simulink model "EffectuatorIntegratedWithDemonstrator"  (R2020a)
settings: Solver=FixedStepDiscrete  StartTime=0.0  StopTime=inf  FixedStep=Ts  RelTol=1e-3
InitFcn:
  | %% Verwende vordefinierte Setpoints (Kreis mit Z-Komponente)
  | 
  | % Config
  | numCircles = 3;
  | scale=6;
  | %Versuch symmetrische Setpunkte zu setzen
  | pointsPerCircle =scale*(4+3*numCircles)+2;
  | 
  | r = 50;
  | m_x = r;
  | m_y = r;
  | 
  | % //
  | s = linspace(0,2*pi,pointsPerCircle);
  | 
  | setPoints_x = [];
  | setPoints_y = [];
  | 
  | for ii=1:numCircles
  | 
  | setPoints_x = [setPoints_x (-cos(s(1:floor(pointsPerCircle / 2))).*r + m_x + 2*r*(ii-1))]; %#ok<AGROW>
  | setPoints_y = [setPoints_y (sin(s).*r+m_y)]; %#ok<AGROW>pointsPerCircle / 2
  | 
  | end
  | 
  | setPoints_x = [setPoints_x flip(setPoints_x(1:end))];
  | 
  | % Loeschen doppelter y-Werte (Kreisuebergang)
  | setPoints_x(pointsPerCircle .* [1:numCircles]) = [];
  | setPoints_y(pointsPerCircle .* [1:numCircles]) = [];
  | 
  | % setPoints_x= [linspace(0,setPoints_x(19),19) setPoints_x(20:end)];
  | % setPoints_y= [linspace(0,setPoints_y(19),19) setPoints_y(20:end)];
  | 
  | % Array Elemente verschieben
  | % setPoints_x = circshift(setPoints_x,-pointsPerCircle/4,2);
  | % setPoints_y = circshift(setPoints_y,-pointsPerCircle/4,2);
  | 
  | z = zeros(1,size(setPoints_x,2));
  | z_x = -5:5;
  | z_y = -z_x.^2 + 25;
  | z_idx = 90;
  | z_idx2 = 210;
  | z(z_idx:z_idx+length(z_x)-1) = z_y;
  | z(z_idx2:z_idx2+length(z_x)-1) = z_y;
  | % z = [z_y z];
  | setPoints_z = z;
  | 
  | % setPoints_x = [zeros(1,length(z_y)) setPoints_x];
  | % setPoints_y = [setPoints_y(1,1)*ones(1,length(z_y)) setPoints_y];
  | 
  | % Umrechnung der Einheiten für Demonstrator
  | % setPoints_x = setPoints_x ./ 1000;
  | % setPoints_y = setPoints_y ./ 1000;
  | % setPoints_z = setPoints_z ./ 1000;
  | 
  | 
  | %{
  | plot(setPoints_x,setPoints_y);
  | fig = figure;
  | ... (+13 lines)
StartFcn:
  | close all;
model workspace (MAT data in the model file):
  MvmtPerfEval_collectVal : Simulink.Parameter (value not decoded)
  MvmtPerfEval_sendOwnVal : Simulink.Parameter (value not decoded)
  PerfEval_numTicks_enable : Simulink.Parameter (value not decoded)
  Segmentregler_I_Gain : Simulink.Parameter (value not decoded)
  Segmentregler_P_Gain : Simulink.Parameter (value not decoded)
  Segmentregler_minVel_enable : Simulink.Parameter (value not decoded)
  Segmentregler_numTicks_enable : Simulink.Parameter (value not decoded)
  Ts : Simulink.Parameter (value not decoded)
  maxPos_x : Simulink.Parameter (value not decoded)
  maxPos_y : Simulink.Parameter (value not decoded)
  maxPos_z : Simulink.Parameter (value not decoded)
  maxVectorLengths : Simulink.Parameter (value not decoded)
  minAllowedVelSaturation : Simulink.Parameter (value not decoded)
  numAxes : Simulink.Parameter (value not decoded)
symbols that are objects in the model workspace (value not decoded): maxPos_x, maxPos_y, maxPos_z, minAllowedVelSaturation, MvmtPerfEval_collectVal, MvmtPerfEval_sendOwnVal, numAxes, PerfEval_numTicks_enable, Segmentregler_I_Gain, Segmentregler_minVel_enable, Segmentregler_numTicks_enable, Segmentregler_P_Gain, Ts
undefined symbols (not defined in the file or in its folder): DiscIntNeverNeededParam, VelOverride
libraries: simulink x20, vrlib x5, sldrtlib x2, xpcrtudplib x2, dspnetwork x2, ptplib x1, etargetslib x1, xpcutilitieslib x1
(part 4 of 5)

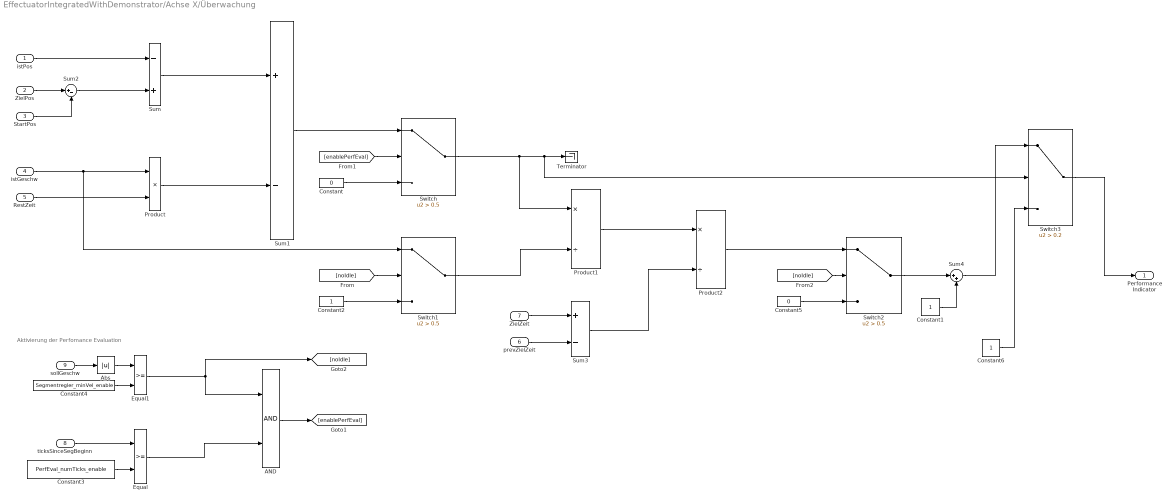
== system EffectuatorIntegratedWithDemonstrator/Achse X/Überwachung ==
  note: Aktivierung der Perfomance Evaluation
  istPos : Inport
  ZielPos : Inport  Port=2
  StartPos : Inport  Port=3
  istGeschw : Inport  Port=4
  RestZeit : Inport  Port=5
  prevZielZeit : Inport  Port=6
  ZielZeit : Inport  Port=7
  ticksSinceSegBeginn : Inport  Port=8
  sollGeschw : Inport  Port=9
  AND : Logic  AllPortsSameDT=off  OutDataTypeStr=boolean
  Abs : Abs
  Constant : Constant  Value=0
  Constant1 : Constant
  Constant2 : Constant
  Constant3 : Constant  Value=PerfEval_numTicks_enable
  Constant4 : Constant  Value=Segmentregler_minVel_enable
  Constant5 : Constant  Value=0
  Constant6 : Constant
  Equal : RelationalOperator  OutDataTypeStr=boolean  RndMeth=Simplest
  Equal1 : RelationalOperator  OutDataTypeStr=boolean  RndMeth=Simplest
  Product : Product
  Product1 : Product  Inputs=*/
  Product2 : Product  Inputs=*/
  Sum : Sum  Inputs=-+
  Sum1 : Sum  Inputs=+-
  Sum2 : Sum  Inputs=|+-
  Sum3 : Sum  Inputs=+-
  Sum4 : Sum  Inputs=|++
  Switch : Switch  Criteria=u2 > Threshold  Threshold=0.5
  Switch1 : Switch  Criteria=u2 > Threshold  Threshold=0.5
  Switch2 : Switch  Criteria=u2 > Threshold  Threshold=0.5
  Switch3 : Switch  Criteria=u2 > Threshold  Threshold=0.2
  Terminator : Terminator
  Performance Indicator : Outport  VectorParamsAs1DForOutWhenUnconnected=off
  wires:
  istPos/1 -> Sum/1
  istGeschw/1 -> Switch1/1, Product/1
  RestZeit/1 -> Product/2
  Product/1 -> Sum1/2
  Sum/1 -> Sum1/1
  ZielPos/1 -> Sum2/1
  StartPos/1 -> Sum2/2
  Sum2/1 -> Sum/2
  Sum1/1 -> Switch/1
  Switch/1 -> Product1/1, Switch3/2, Terminator/1
  [enablePerfEval] -> Switch/2
  Constant/1 -> Switch/3
  Product1/1 -> Product2/1
  Sum3/1 -> Product2/2
  prevZielZeit/1 -> Sum3/2
  ZielZeit/1 -> Sum3/1
  Sum4/1 -> Switch3/1
  Constant1/1 -> Sum4/2
  ticksSinceSegBeginn/1 -> Equal/1
  Constant3/1 -> Equal/2
  Equal/1 -> AND/2
  sollGeschw/1 -> Abs/1
  Constant4/1 -> Equal1/2
  Equal1/1 -> [noIdle], AND/1
  AND/1 -> [enablePerfEval]
  [noIdle] -> Switch1/2
  Constant2/1 -> Switch1/3
  Switch1/1 -> Product1/2
  Switch2/1 -> Sum4/1
  Product2/1 -> Switch2/1
  [noIdle] -> Switch2/2
  Constant5/1 -> Switch2/3
  Abs/1 -> Equal1/1
  Switch3/1 -> Performance Indicator/1
  Constant6/1 -> Switch3/3

== system EffectuatorIntegratedWithDemonstrator/Achse Y/Sat_maxGeschw ==
  Threshold : Inport
  In : Inport  Port=2
  Threshold1 : Inport  Port=3
  Abs : Abs
  Constant : Constant  Value=0
  Multiply : Gain  Gain=-1
  Sign : Signum
  Sum3 : Sum  Inputs=-+
  Switch : Switch  Criteria=u2 > Threshold
  Switch1 : Switch
  Switch2 : Switch  Criteria=u2 > Threshold
  Out : Outport  VectorParamsAs1DForOutWhenUnconnected=off
  wires:
  Sum3/1 -> Switch/2
  Threshold/1 -> Switch/1, Sum3/1
  Abs/1 -> Sum3/2, Switch/3
  In/1 -> Sign/1, Abs/1
  Sign/1 -> Switch1/2
  Switch/1 -> Multiply/1, Switch1/1
  Multiply/1 -> Switch1/3
  Switch2/1 -> Out/1
  Constant/1 -> Switch2/3
  Threshold1/1 -> Switch2/2
  Switch1/1 -> Switch2/1

== system EffectuatorIntegratedWithDemonstrator/Achse Y/Sat_sollGeschw ==
  Threshold : Inport
  In : Inport  Port=2
  Abs : Abs
  Constant : Constant  Value=minAllowedVelSaturation
  Max : MinMax  Function=max  Inputs=2
  Multiply : Gain  Gain=-1
  Sign : Signum
  Sum3 : Sum  Inputs=-+
  Switch : Switch  Criteria=u2 > Threshold
  Switch1 : Switch
  Out : Outport  VectorParamsAs1DForOutWhenUnconnected=off
  wires:
  Constant/1 -> Max/2
  Threshold/1 -> Max/1
  Switch1/1 -> Out/1
  Multiply/1 -> Switch1/3
  Switch/1 -> Switch1/1, Multiply/1
  Sign/1 -> Switch1/2
  In/1 -> Abs/1, Sign/1
  Abs/1 -> Switch/3, Sum3/2
  Max/1 -> Sum3/1, Switch/1
  Sum3/1 -> Switch/2

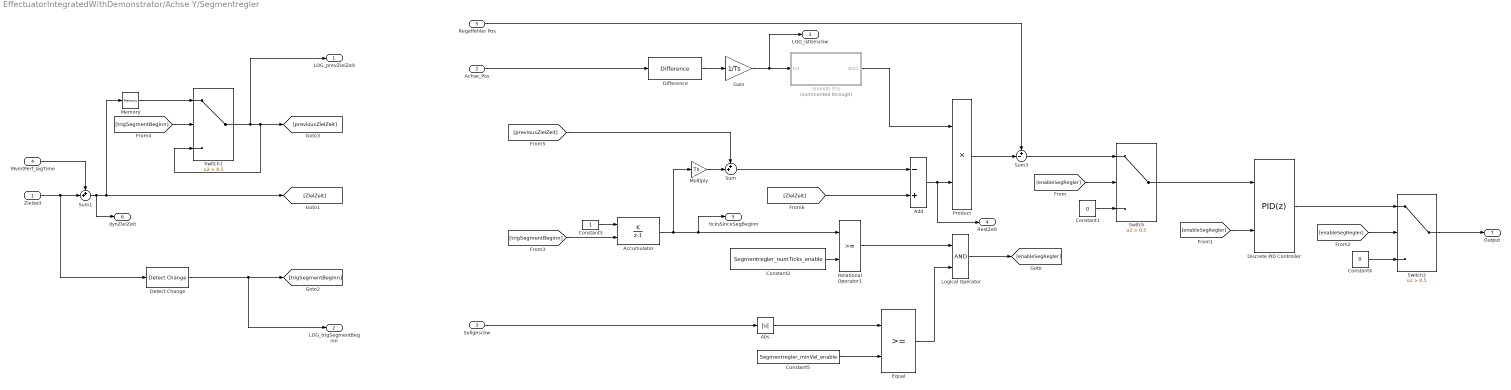
== system EffectuatorIntegratedWithDemonstrator/Achse Y/Segmentregler ==
  Zielzeit : Inport
  Achse_Pos : Inport  Port=2
  Sollgeschw : Inport  Port=3
  MvmtPerf_lagTime : Inport  Port=4
  Regelfehler Pos : Inport  Port=5
  Abs : Abs
  Accumulator : DiscreteIntegrator  IntegratorMethod=Accumulation: Forward Euler  gainval=1  ExternalReset=rising  SampleTime=-1  ICPrevOutput=DiscIntNeverNeededParam  ICPrevScaledInput=DiscIntNeverNeededParam
  Add : Sum  Inputs=-+
  Constant1 : Constant  Value=0
  Constant2 : Constant  Value=Segmentregler_numTicks_enable
  Constant3 : Constant
  Constant4 : Constant  Value=0
  Constant5 : Constant  Value=Segmentregler_minVel_enable
  Detect Change : simulink/Logic and Bit Operations/Detect Change  vinit=0  OutDataTypeStr=boolean
  Difference : simulink/Discrete/Difference  ICPrevInput=0.0  OutMin=[]  OutMax=[]  OutDataType=fixdt(1, 16)  OutScaling=2^-10  DoSatur=off
  Discrete PID Controller : simulink/Continuous/PID Controller  Controller=PID  Form=Parallel  TimeDomain=Discrete-time  UseExternalTs=off  SampleTime=-1  IntegratorMethod=Forward Euler  FilterMethod=Forward Euler  ControllerParametersSource=internal  P=Segmentregler_P_Gain  I=Segmentregler_I_Gain  D=0  UseFilter=on  N=100  TunerSelectOption=Transfer Function Based (PID Tuner App)  InitialConditionSource=internal  InitialConditionForIntegrator=0  InitialConditionForFilter=0  DifferentiatorICPrevScaledInput=0  ExternalReset=falling  TrackingMode=off  Kt=1  LimitOutput=off  UpperSaturationLimit=inf  LowerSaturationLimit=-inf  LinearizeAsGain=off  AntiWindupMode=none  Kb=1  POutMin=[]  POutMax=[]  IOutMin=[]  IOutMax=[]  DOutMin=[]  DOutMax=[]  NOutMin=[]  NOutMax=[]  SumOutMin=[]  SumOutMax=[]  SaturationOutMin=[]  SaturationOutMax=[]  PParamMin=[]  PParamMax=[]  IParamMin=[]  IParamMax=[]  DParamMin=[]  DParamMax=[]  NParamMin=[]  NParamMax=[]  KbParamMin=[]  KbParamMax=[]  KtParamMin=[]  KtParamMax=[]  KbOutMin=[]  KbOutMax=[]  KtOutMin=[]  KtOutMax=[]  IntegratorOutMin=[]  IntegratorOutMax=[]  FilterOutMin=[]  FilterOutMax=[]  SumI1OutMin=[]  SumI1OutMax=[]  SumI2OutMin=[]  SumI2OutMax=[]  SumI3OutMin=[]  SumI3OutMax=[]  SumI4OutMin=[]  SumI4OutMax=[]  SumDOutMin=[]  SumDOutMax=[]  DifferentiatorOutMin=[]  DifferentiatorOutMax=[]  FilterDiffOutCoefMin=[]  FilterDiffOutCoefMax=[]  ReciprocalOutMin=[]  ReciprocalOutMax=[]  SumDenOutMin=[]  SumDenOutMax=[]  SumNumOutMin=[]  SumNumOutMax=[]  DivideOutMin=[]  DivideOutMax=[]  UdiffTsProdOutMin=[]  UdiffTsProdOutMax=[]  NTsProdOutMin=[]  NTsProdOutMax=[]  UintegralTsProdOutMin=[]  UintegralTsProdOutMax=[]  UngainTsProdOutMin=[]  UngainTsProdOutMax=[]  IntegratorContinuousStateAttributes=''  IntegratorStateMustResolveToSignalObject=off  IntegratorRTWStateStorageClass=Auto  FilterContinuousStateAttributes=''  FilterStateMustResolveToSignalObject=off  FilterRTWStateStorageClass=Auto  ParallelPVariant=InternalParameters  IdealPVariant=Disabled  IVariant=InternalParameters  DVariant=InternalParameters  IntegratorVariant=Discrete  SatVariant=Disabled  AWVariant=Passthrough  PCopyVariant=Disabled  TRVariant=Disabled  FdbkBlocksVariant=Forward  IdealPFdbkVariant=Disabled  SatFdbkVariant=Disabled  DerivativeFilterVariant=ForwardEulerFilter  NVariant=InternalParameters  NCopyVariant=Disabled  FilterICVariant=InternalICsFilter  IntegratorICVariant=InternalICs  ExternalResetVariant=ExternalReset  TRSumVariant=Passthrough  SumFdbkVariant=Disabled  SumVariant=Sum_PID  TsampFilterVariant=InternalTs  TsampNgainVariant=Passthrough  TsampIntegralVariant=Passthrough
  Equal : RelationalOperator  OutDataTypeStr=boolean  RndMeth=Simplest
  Gain : Gain  Gain=1/Ts
  Logical Operator : Logic  AllPortsSameDT=off  OutDataTypeStr=boolean
  Memory : Memory
  Multiply : Gain  Gain=Ts
  Product : Product
  Relational Operator1 : RelationalOperator  OutDataTypeStr=boolean  RndMeth=Simplest
  Smooth 5Ts : Subsystem  Commented=through
  Sum : Sum  Inputs=++|
  Sum1 : Sum  Inputs=++|
  Sum3 : Sum  Inputs=+-|
  Switch : Switch  Criteria=u2 > Threshold  Threshold=0.5
  Switch1 : Switch  Criteria=u2 > Threshold  Threshold=0.5
  Switch2 : Switch  Criteria=u2 > Threshold  Threshold=0.5
  LOG_prevZielZeit : Outport  VectorParamsAs1DForOutWhenUnconnected=off
  LOG_trigSegmentBeginn : Outport  Port=2  VectorParamsAs1DForOutWhenUnconnected=off
  LOG_istGeschw : Outport  Port=3  VectorParamsAs1DForOutWhenUnconnected=off
  RestZeit : Outport  Port=4  VectorParamsAs1DForOutWhenUnconnected=off
  ticksSinceSegBeginn : Outport  Port=5  VectorParamsAs1DForOutWhenUnconnected=off
  dynZielZeit : Outport  Port=6  VectorParamsAs1DForOutWhenUnconnected=off
  Output : Outport  Port=7  VectorParamsAs1DForOutWhenUnconnected=off
  wires:
  MvmtPerf_lagTime/1 -> Sum1/1
  Zielzeit/1 -> Sum1/2, Detect Change/1
  Abs/1 -> Equal/1
  Sum1/1 -> [ZielZeit], Memory/1, dynZielZeit/1
  [ZielZeit] -> Add/2
  Multiply/1 -> Sum/2
  Smooth 5Ts/1(Out1) -> Product/1
  [previousZielZeit] -> Sum/1
  Switch1/1 -> [previousZielZeit], Switch1/3, LOG_prevZielZeit/1
  [trigSegmentBeginn] -> Switch1/2
  [trigSegmentBeginn] -> Accumulator/2
  Detect Change/1 -> [trigSegmentBeginn], LOG_trigSegmentBeginn/1
  Gain/1 -> Smooth 5Ts/1(In1), LOG_istGeschw/1
  Memory/1 -> Switch1/1
  Equal/1 -> Logical Operator/2
  Constant5/1 -> Equal/2
  Sollgeschw/1 -> Abs/1
  [enableSegRegler] -> Switch2/2
  [enableSegRegler] -> Discrete PID Controller/2
  [enableSegRegler] -> Switch/2
  Logical Operator/1 -> [enableSegRegler]
  Switch2/1 -> Output/1
  Regelfehler Pos/1 -> Sum3/1
  Product/1 -> Sum3/2
  Constant4/1 -> Switch2/3
  Constant1/1 -> Switch/3
  Discrete PID Controller/1 -> Switch2/1
  Achse_Pos/1 -> Difference/1
  Constant2/1 -> Relational Operator1/2
  Add/1 -> Product/2, RestZeit/1
  Relational Operator1/1 -> Logical Operator/1
  Sum/1 -> Add/1
  Switch/1 -> Discrete PID Controller/1
  Sum3/1 -> Switch/1
  Difference/1 -> Gain/1
  Accumulator/1 -> Relational Operator1/1, ticksSinceSegBeginn/1, Multiply/1
  Constant3/1 -> Accumulator/1

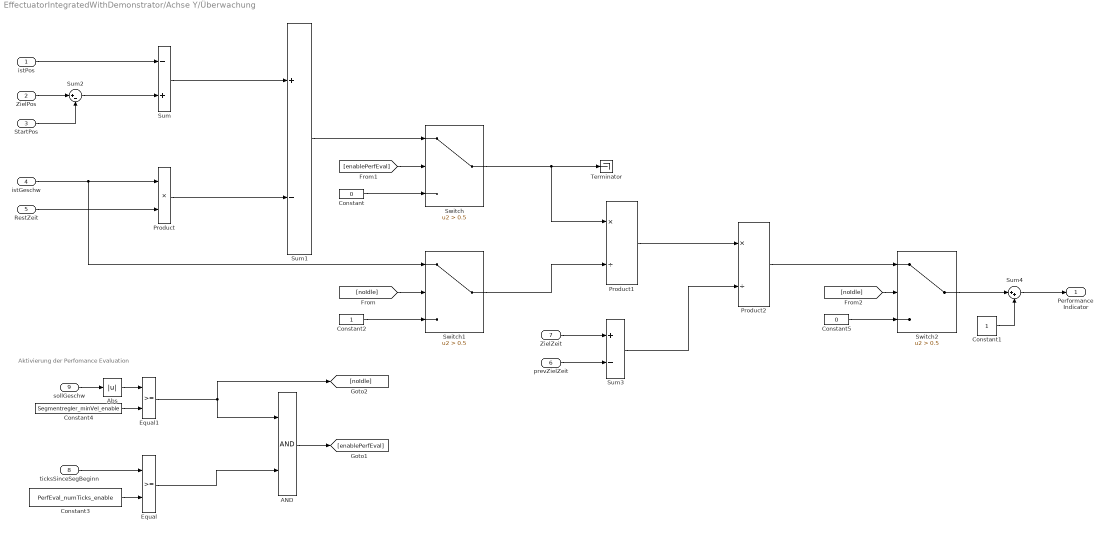
== system EffectuatorIntegratedWithDemonstrator/Achse Y/Überwachung ==
  note: Aktivierung der Perfomance Evaluation
  istPos : Inport
  ZielPos : Inport  Port=2
  StartPos : Inport  Port=3
  istGeschw : Inport  Port=4
  RestZeit : Inport  Port=5
  prevZielZeit : Inport  Port=6
  ZielZeit : Inport  Port=7
  ticksSinceSegBeginn : Inport  Port=8
  sollGeschw : Inport  Port=9
  AND : Logic  AllPortsSameDT=off  OutDataTypeStr=boolean
  Abs : Abs
  Constant : Constant  Value=0
  Constant1 : Constant
  Constant2 : Constant
  Constant3 : Constant  Value=PerfEval_numTicks_enable
  Constant4 : Constant  Value=Segmentregler_minVel_enable
  Constant5 : Constant  Value=0
  Equal : RelationalOperator  OutDataTypeStr=boolean  RndMeth=Simplest
  Equal1 : RelationalOperator  OutDataTypeStr=boolean  RndMeth=Simplest
  Product : Product
  Product1 : Product  Inputs=*/
  Product2 : Product  Inputs=*/
  Sum : Sum  Inputs=-+
  Sum1 : Sum  Inputs=+-
  Sum2 : Sum  Inputs=|+-
  Sum3 : Sum  Inputs=+-
  Sum4 : Sum  Inputs=|++
  Switch : Switch  Criteria=u2 > Threshold  Threshold=0.5
  Switch1 : Switch  Criteria=u2 > Threshold  Threshold=0.5
  Switch2 : Switch  Criteria=u2 > Threshold  Threshold=0.5
  Terminator : Terminator
  Performance Indicator : Outport  VectorParamsAs1DForOutWhenUnconnected=off
  wires:
  Abs/1 -> Equal1/1
  Constant5/1 -> Switch2/3
  [noIdle] -> Switch2/2
  Product2/1 -> Switch2/1
  Switch2/1 -> Sum4/1
  Switch1/1 -> Product1/2
  Constant2/1 -> Switch1/3
  [noIdle] -> Switch1/2
  AND/1 -> [enablePerfEval]
  Equal1/1 -> AND/1, [noIdle]
  Constant4/1 -> Equal1/2
  sollGeschw/1 -> Abs/1
  Equal/1 -> AND/2
  Constant3/1 -> Equal/2
  ticksSinceSegBeginn/1 -> Equal/1
  Constant1/1 -> Sum4/2
  Sum4/1 -> Performance Indicator/1
  ZielZeit/1 -> Sum3/1
  prevZielZeit/1 -> Sum3/2
  Sum3/1 -> Product2/2
  Product1/1 -> Product2/1
  Constant/1 -> Switch/3
  [enablePerfEval] -> Switch/2
  Switch/1 -> Terminator/1, Product1/1
  Sum1/1 -> Switch/1
  Sum2/1 -> Sum/2
  StartPos/1 -> Sum2/2
  ZielPos/1 -> Sum2/1
  Sum/1 -> Sum1/1
  Product/1 -> Sum1/2
  RestZeit/1 -> Product/2
  istGeschw/1 -> Product/1, Switch1/1
  istPos/1 -> Sum/1

== system EffectuatorIntegratedWithDemonstrator/Achse Z/Sat_maxGeschw ==
  Threshold : Inport
  In : Inport  Port=2
  Threshold1 : Inport  Port=3
  Abs : Abs
  Constant : Constant  Value=0
  Multiply : Gain  Gain=-1
  Sign : Signum
  Sum3 : Sum  Inputs=-+
  Switch : Switch  Criteria=u2 > Threshold
  Switch1 : Switch
  Switch2 : Switch  Criteria=u2 > Threshold
  Out : Outport  VectorParamsAs1DForOutWhenUnconnected=off
  wires:
  Multiply/1 -> Switch1/3
  Switch/1 -> Switch1/1, Multiply/1
  Sign/1 -> Switch1/2
  In/1 -> Abs/1, Sign/1
  Abs/1 -> Switch/3, Sum3/2
  Threshold/1 -> Sum3/1, Switch/1
  Sum3/1 -> Switch/2
  Switch2/1 -> Out/1
  Switch1/1 -> Switch2/1
  Constant/1 -> Switch2/3
  Threshold1/1 -> Switch2/2

== system EffectuatorIntegratedWithDemonstrator/Achse Z/Sat_sollGeschw ==
  Threshold : Inport
  In : Inport  Port=2
  Abs : Abs
  Constant : Constant  Value=minAllowedVelSaturation
  Max : MinMax  Function=max  Inputs=2
  Multiply : Gain  Gain=-1
  Sign : Signum
  Sum3 : Sum  Inputs=-+
  Switch : Switch  Criteria=u2 > Threshold
  Switch1 : Switch
  Out : Outport  VectorParamsAs1DForOutWhenUnconnected=off
  wires:
  Sum3/1 -> Switch/2
  Max/1 -> Switch/1, Sum3/1
  Abs/1 -> Sum3/2, Switch/3
  In/1 -> Sign/1, Abs/1
  Sign/1 -> Switch1/2
  Switch/1 -> Multiply/1, Switch1/1
  Multiply/1 -> Switch1/3
  Switch1/1 -> Out/1
  Threshold/1 -> Max/1
  Constant/1 -> Max/2

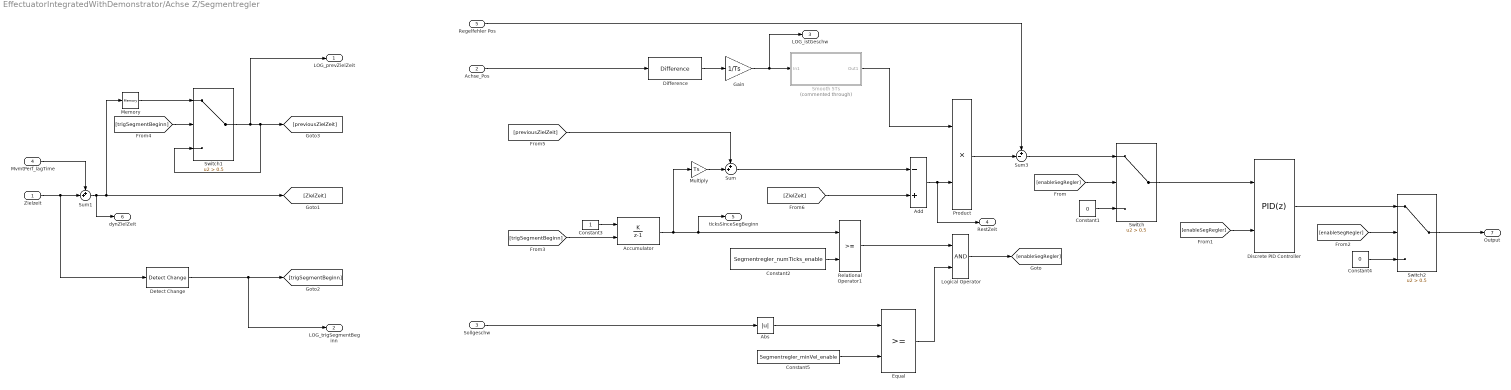
== system EffectuatorIntegratedWithDemonstrator/Achse Z/Segmentregler ==
  Zielzeit : Inport
  Achse_Pos : Inport  Port=2
  Sollgeschw : Inport  Port=3
  MvmtPerf_lagTime : Inport  Port=4
  Regelfehler Pos : Inport  Port=5
  Abs : Abs
  Accumulator : DiscreteIntegrator  IntegratorMethod=Accumulation: Forward Euler  gainval=1  ExternalReset=rising  SampleTime=-1  ICPrevOutput=DiscIntNeverNeededParam  ICPrevScaledInput=DiscIntNeverNeededParam
  Add : Sum  Inputs=-+
  Constant1 : Constant  Value=0
  Constant2 : Constant  Value=Segmentregler_numTicks_enable
  Constant3 : Constant
  Constant4 : Constant  Value=0
  Constant5 : Constant  Value=Segmentregler_minVel_enable
  Detect Change : simulink/Logic and Bit Operations/Detect Change  vinit=0  OutDataTypeStr=boolean
  Difference : simulink/Discrete/Difference  ICPrevInput=0.0  OutMin=[]  OutMax=[]  OutDataType=fixdt(1, 16)  OutScaling=2^-10  DoSatur=off
  Discrete PID Controller : simulink/Continuous/PID Controller  Controller=PID  Form=Parallel  TimeDomain=Discrete-time  UseExternalTs=off  SampleTime=-1  IntegratorMethod=Forward Euler  FilterMethod=Forward Euler  ControllerParametersSource=internal  P=Segmentregler_P_Gain  I=Segmentregler_I_Gain  D=0  UseFilter=on  N=100  TunerSelectOption=Transfer Function Based (PID Tuner App)  InitialConditionSource=internal  InitialConditionForIntegrator=0  InitialConditionForFilter=0  DifferentiatorICPrevScaledInput=0  ExternalReset=falling  TrackingMode=off  Kt=1  LimitOutput=off  UpperSaturationLimit=inf  LowerSaturationLimit=-inf  LinearizeAsGain=off  AntiWindupMode=none  Kb=1  POutMin=[]  POutMax=[]  IOutMin=[]  IOutMax=[]  DOutMin=[]  DOutMax=[]  NOutMin=[]  NOutMax=[]  SumOutMin=[]  SumOutMax=[]  SaturationOutMin=[]  SaturationOutMax=[]  PParamMin=[]  PParamMax=[]  IParamMin=[]  IParamMax=[]  DParamMin=[]  DParamMax=[]  NParamMin=[]  NParamMax=[]  KbParamMin=[]  KbParamMax=[]  KtParamMin=[]  KtParamMax=[]  KbOutMin=[]  KbOutMax=[]  KtOutMin=[]  KtOutMax=[]  IntegratorOutMin=[]  IntegratorOutMax=[]  FilterOutMin=[]  FilterOutMax=[]  SumI1OutMin=[]  SumI1OutMax=[]  SumI2OutMin=[]  SumI2OutMax=[]  SumI3OutMin=[]  SumI3OutMax=[]  SumI4OutMin=[]  SumI4OutMax=[]  SumDOutMin=[]  SumDOutMax=[]  DifferentiatorOutMin=[]  DifferentiatorOutMax=[]  FilterDiffOutCoefMin=[]  FilterDiffOutCoefMax=[]  ReciprocalOutMin=[]  ReciprocalOutMax=[]  SumDenOutMin=[]  SumDenOutMax=[]  SumNumOutMin=[]  SumNumOutMax=[]  DivideOutMin=[]  DivideOutMax=[]  UdiffTsProdOutMin=[]  UdiffTsProdOutMax=[]  NTsProdOutMin=[]  NTsProdOutMax=[]  UintegralTsProdOutMin=[]  UintegralTsProdOutMax=[]  UngainTsProdOutMin=[]  UngainTsProdOutMax=[]  IntegratorContinuousStateAttributes=''  IntegratorStateMustResolveToSignalObject=off  IntegratorRTWStateStorageClass=Auto  FilterContinuousStateAttributes=''  FilterStateMustResolveToSignalObject=off  FilterRTWStateStorageClass=Auto  ParallelPVariant=InternalParameters  IdealPVariant=Disabled  IVariant=InternalParameters  DVariant=InternalParameters  IntegratorVariant=Discrete  SatVariant=Disabled  AWVariant=Passthrough  PCopyVariant=Disabled  TRVariant=Disabled  FdbkBlocksVariant=Forward  IdealPFdbkVariant=Disabled  SatFdbkVariant=Disabled  DerivativeFilterVariant=ForwardEulerFilter  NVariant=InternalParameters  NCopyVariant=Disabled  FilterICVariant=InternalICsFilter  IntegratorICVariant=InternalICs  ExternalResetVariant=ExternalReset  TRSumVariant=Passthrough  SumFdbkVariant=Disabled  SumVariant=Sum_PID  TsampFilterVariant=InternalTs  TsampNgainVariant=Passthrough  TsampIntegralVariant=Passthrough
  Equal : RelationalOperator  OutDataTypeStr=boolean  RndMeth=Simplest
  Gain : Gain  Gain=1/Ts
  Logical Operator : Logic  AllPortsSameDT=off  OutDataTypeStr=boolean
  Memory : Memory
  Multiply : Gain  Gain=Ts
  Product : Product
  Relational Operator1 : RelationalOperator  OutDataTypeStr=boolean  RndMeth=Simplest
  Smooth 5Ts : Subsystem  Commented=through
  Sum : Sum  Inputs=++|
  Sum1 : Sum  Inputs=++|
  Sum3 : Sum  Inputs=+-|
  Switch : Switch  Criteria=u2 > Threshold  Threshold=0.5
  Switch1 : Switch  Criteria=u2 > Threshold  Threshold=0.5
  Switch2 : Switch  Criteria=u2 > Threshold  Threshold=0.5
  LOG_prevZielZeit : Outport  VectorParamsAs1DForOutWhenUnconnected=off
  LOG_trigSegmentBeginn : Outport  Port=2  VectorParamsAs1DForOutWhenUnconnected=off
  LOG_istGeschw : Outport  Port=3  VectorParamsAs1DForOutWhenUnconnected=off
  RestZeit : Outport  Port=4  VectorParamsAs1DForOutWhenUnconnected=off
  ticksSinceSegBeginn : Outport  Port=5  VectorParamsAs1DForOutWhenUnconnected=off
  dynZielZeit : Outport  Port=6  VectorParamsAs1DForOutWhenUnconnected=off
  Output : Outport  Port=7  VectorParamsAs1DForOutWhenUnconnected=off
  wires:
  Constant3/1 -> Accumulator/1
  Accumulator/1 -> Multiply/1, ticksSinceSegBeginn/1, Relational Operator1/1
  Difference/1 -> Gain/1
  Sum3/1 -> Switch/1
  Switch/1 -> Discrete PID Controller/1
  Sum/1 -> Add/1
  Relational Operator1/1 -> Logical Operator/1
  Add/1 -> RestZeit/1, Product/2
  Constant2/1 -> Relational Operator1/2
  Achse_Pos/1 -> Difference/1
  Discrete PID Controller/1 -> Switch2/1
  Constant1/1 -> Switch/3
  Constant4/1 -> Switch2/3
  Product/1 -> Sum3/2
  Regelfehler Pos/1 -> Sum3/1
  Switch2/1 -> Output/1
  Logical Operator/1 -> [enableSegRegler]
  [enableSegRegler] -> Switch/2
  [enableSegRegler] -> Discrete PID Controller/2
  [enableSegRegler] -> Switch2/2
  Sollgeschw/1 -> Abs/1
  Constant5/1 -> Equal/2
  Equal/1 -> Logical Operator/2
  Memory/1 -> Switch1/1
  Gain/1 -> LOG_istGeschw/1, Smooth 5Ts/1(In1)
  Detect Change/1 -> LOG_trigSegmentBeginn/1, [trigSegmentBeginn]
  [trigSegmentBeginn] -> Accumulator/2
  [trigSegmentBeginn] -> Switch1/2
  Switch1/1 -> LOG_prevZielZeit/1, Switch1/3, [previousZielZeit]
  [previousZielZeit] -> Sum/1
  Smooth 5Ts/1(Out1) -> Product/1
  Multiply/1 -> Sum/2
  [ZielZeit] -> Add/2
  Sum1/1 -> dynZielZeit/1, Memory/1, [ZielZeit]
  Abs/1 -> Equal/1
  Zielzeit/1 -> Detect Change/1, Sum1/2
  MvmtPerf_lagTime/1 -> Sum1/1

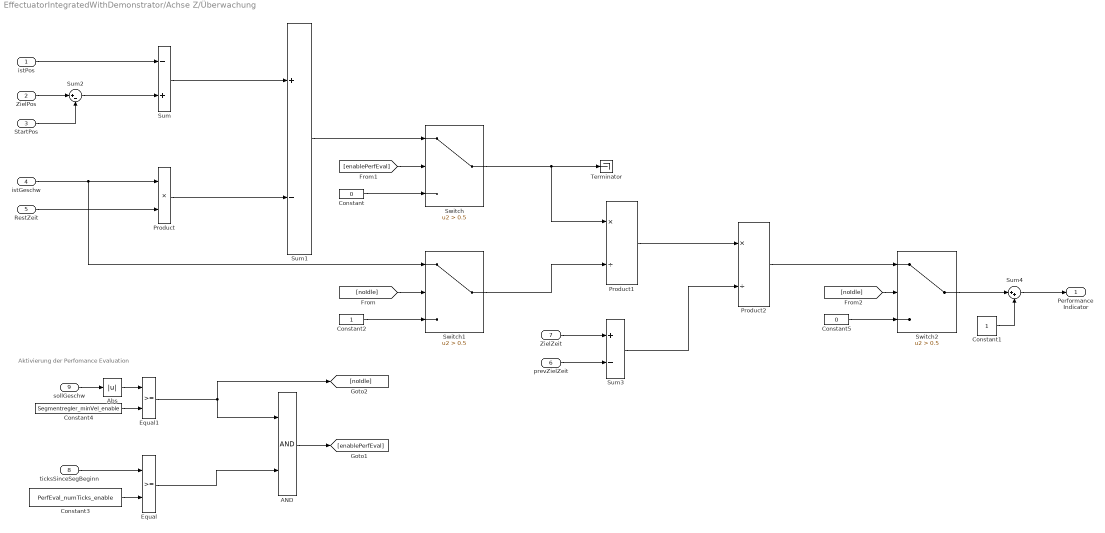
== system EffectuatorIntegratedWithDemonstrator/Achse Z/Überwachung ==
  note: Aktivierung der Perfomance Evaluation
  istPos : Inport
  ZielPos : Inport  Port=2
  StartPos : Inport  Port=3
  istGeschw : Inport  Port=4
  RestZeit : Inport  Port=5
  prevZielZeit : Inport  Port=6
  ZielZeit : Inport  Port=7
  ticksSinceSegBeginn : Inport  Port=8
  sollGeschw : Inport  Port=9
  AND : Logic  AllPortsSameDT=off  OutDataTypeStr=boolean
  Abs : Abs
  Constant : Constant  Value=0
  Constant1 : Constant
  Constant2 : Constant
  Constant3 : Constant  Value=PerfEval_numTicks_enable
  Constant4 : Constant  Value=Segmentregler_minVel_enable
  Constant5 : Constant  Value=0
  Equal : RelationalOperator  OutDataTypeStr=boolean  RndMeth=Simplest
  Equal1 : RelationalOperator  OutDataTypeStr=boolean  RndMeth=Simplest
  Product : Product
  Product1 : Product  Inputs=*/
  Product2 : Product  Inputs=*/
  Sum : Sum  Inputs=-+
  Sum1 : Sum  Inputs=+-
  Sum2 : Sum  Inputs=|+-
  Sum3 : Sum  Inputs=+-
  Sum4 : Sum  Inputs=|++
  Switch : Switch  Criteria=u2 > Threshold  Threshold=0.5
  Switch1 : Switch  Criteria=u2 > Threshold  Threshold=0.5
  Switch2 : Switch  Criteria=u2 > Threshold  Threshold=0.5
  Terminator : Terminator
  Performance Indicator : Outport  VectorParamsAs1DForOutWhenUnconnected=off
  wires:
  istPos/1 -> Sum/1
  istGeschw/1 -> Switch1/1, Product/1
  RestZeit/1 -> Product/2
  Product/1 -> Sum1/2
  Sum/1 -> Sum1/1
  ZielPos/1 -> Sum2/1
  StartPos/1 -> Sum2/2
  Sum2/1 -> Sum/2
  Sum1/1 -> Switch/1
  Switch/1 -> Product1/1, Terminator/1
  [enablePerfEval] -> Switch/2
  Constant/1 -> Switch/3
  Product1/1 -> Product2/1
  Sum3/1 -> Product2/2
  prevZielZeit/1 -> Sum3/2
  ZielZeit/1 -> Sum3/1
  Sum4/1 -> Performance Indicator/1
  Constant1/1 -> Sum4/2
  ticksSinceSegBeginn/1 -> Equal/1
  Constant3/1 -> Equal/2
  Equal/1 -> AND/2
  sollGeschw/1 -> Abs/1
  Constant4/1 -> Equal1/2
  Equal1/1 -> [noIdle], AND/1
  AND/1 -> [enablePerfEval]
  [noIdle] -> Switch1/2
  Constant2/1 -> Switch1/3
  Switch1/1 -> Product1/2
  Switch2/1 -> Sum4/1
  Product2/1 -> Switch2/1
  [noIdle] -> Switch2/2
  Constant5/1 -> Switch2/3
  Abs/1 -> Equal1/1

== system EffectuatorIntegratedWithDemonstrator/Joystick Ctrl/Fetch_Global_Data ==
  Chart : Stateflow chart  TreatAsAtomicUnit=on  SystemSampleTime=0.2
  Mux : Mux  Inputs=6
  Terminator : Terminator
  wires:
  Chart/2(velOR_y) -> Mux/2
  Chart/1(velOR_x) -> Mux/1
  Chart/6(vel_z) -> Mux/6
  Chart/4(vel_x) -> Mux/4
  Chart/5(vel_y) -> Mux/5
  Chart/3(velOR_z) -> Mux/3
  Mux/1 -> Terminator/1

== system EffectuatorIntegratedWithDemonstrator/Joystick Ctrl/Joystick ==
  AchseX : Subsystem
  AchseY : Subsystem
  AchseZ : Subsystem
  Bus Creator : BusCreator  Inputs=2
  Joystick Input : vrlib/Joystick Input  joyid=1  adjustports=off  forcefeed=off
  wires:
  Joystick Input/2 -> Bus Creator/2
  Joystick Input/1 -> Bus Creator/1
  Bus Creator/1 -> AchseZ/1(Inport), AchseX/1(Inport), AchseY/1(Inport)

== system EffectuatorIntegratedWithDemonstrator/Joystick Ctrl/Sliders ==
  Constant : Constant
  Constant1 : Constant
  Constant2 : Constant
  Constant3 : Constant  Value=0.125
  Constant4 : Constant  Value=0.125
  Constant5 : Constant  Value=0.125
  Data Store Write : DataStoreWrite  DataStoreName=VelOverride  SampleTime=0.5  DataStoreElements=VelOverride(1)
  Data Store Write1 : DataStoreWrite  DataStoreName=VelOverride  SampleTime=0.5  DataStoreElements=VelOverride(2)
  Data Store Write2 : DataStoreWrite  DataStoreName=VelOverride  SampleTime=0.5  DataStoreElements=VelOverride(3)
  Min : MinMax  Function=max  Inputs=2
  Min1 : MinMax  Function=max  Inputs=2
  Min2 : MinMax  Function=max  Inputs=2
  wires:
  Constant3/1 -> Min/1
  Constant/1 -> Min/2
  Min/1 -> Data Store Write/1
  Constant4/1 -> Min1/1
  Constant1/1 -> Min1/2
  Min1/1 -> Data Store Write1/1
  Constant5/1 -> Min2/1
  Constant2/1 -> Min2/2
  Min2/1 -> Data Store Write2/1

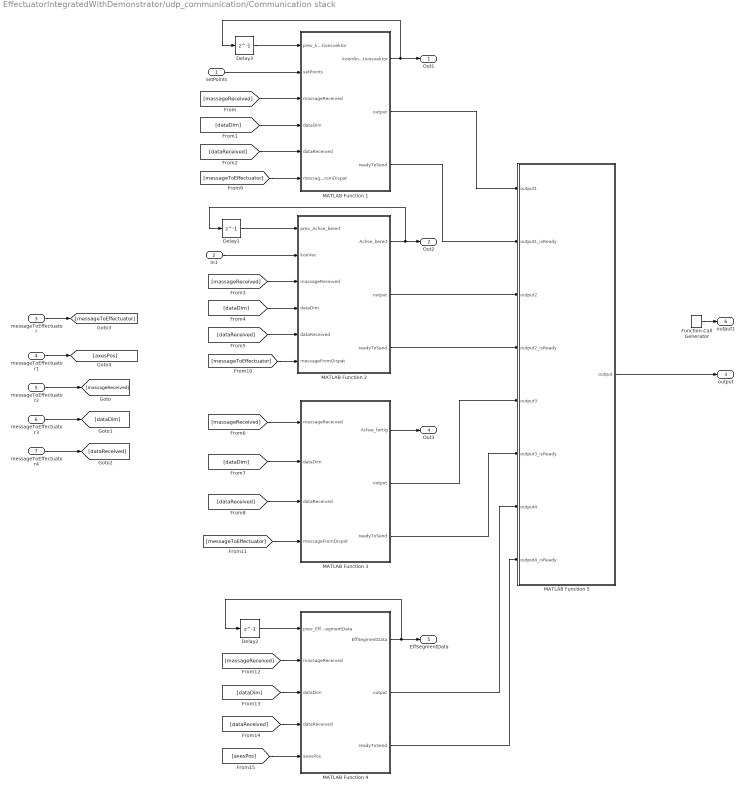
== system EffectuatorIntegratedWithDemonstrator/udp_communication/Communication stack ==
  setPoints : Inport
  In1 : Inport  Port=2
  messageToEffectuator : Inport  Port=3
  messageToEffectuator1 : Inport  Port=4
  messageToEffectuator2 : Inport  Port=5
  messageToEffectuator3 : Inport  Port=6
  messageToEffectuator4 : Inport  Port=7
  Delay1 : Delay  DelayLength=1
  Delay2 : Delay  DelayLength=1
  Delay3 : Delay  DelayLength=1
  Function-Call Generator : simulink/Ports & Subsystems/Function-Call Generator  sample_time=1  numberOfIterations=1
  "MATLAB Function 1 " : MATLAB Function  TreatAsAtomicUnit=on
  MATLAB Function 2 : MATLAB Function  TreatAsAtomicUnit=on
  MATLAB Function 3 : MATLAB Function  TreatAsAtomicUnit=on
  MATLAB Function 4 : MATLAB Function  TreatAsAtomicUnit=on
  MATLAB Function 5 : MATLAB Function  TreatAsAtomicUnit=on
  Out1 : Outport
  Out2 : Outport  Port=2
  output : Outport  Port=3
  Out3 : Outport  Port=4
  EffSegmentData : Outport  Port=5
  output1 : Outport  Port=6
  wires:
  Delay3/1 -> "MATLAB Function 1 "/1(prev_koordinationsvektor)
  [dataReceived] -> MATLAB Function 2/5(dataReceived)
  [massageReceived] -> MATLAB Function 3/1(massageReceived)
  [dataReceived] -> "MATLAB Function 1 "/5(dataReceived)
  MATLAB Function 2/3(readyToSend) -> MATLAB Function 5/4(output2_isReady)
  [massageReceived] -> MATLAB Function 2/3(massageReceived)
  [axesPos] -> MATLAB Function 4/5(axesPos)
  [dataReceived] -> MATLAB Function 3/3(dataReceived)
  "MATLAB Function 1 "/1(koordinationsvektor) -> Out1/1, Delay3/1
  MATLAB Function 3/2(output) -> MATLAB Function 5/5(output3)
  [messageToEffectuator] -> MATLAB Function 2/6(messageFromDispat)
  MATLAB Function 2/2(output) -> MATLAB Function 5/3(output2)
  [messageToEffectuator] -> "MATLAB Function 1 "/6(messageFromDispat)
  setPoints/1 -> "MATLAB Function 1 "/2(setPoints)
  MATLAB Function 4/1(EffSegmentData) -> EffSegmentData/1, Delay2/1
  MATLAB Function 3/3(readyToSend) -> MATLAB Function 5/6(output3_isReady)
  Delay1/1 -> MATLAB Function 2/1(prev_Achse_bereit)
  MATLAB Function 2/1(Achse_bereit) -> Out2/1, Delay1/1
  [dataDim] -> MATLAB Function 2/4(dataDim)
  "MATLAB Function 1 "/2(output) -> MATLAB Function 5/1(output1)
  "MATLAB Function 1 "/3(readyToSend) -> MATLAB Function 5/2(output1_isReady)
  [dataDim] -> MATLAB Function 3/2(dataDim)
  [massageReceived] -> MATLAB Function 4/2(massageReceived)
  MATLAB Function 3/1(Achse_fertig) -> Out3/1
  [dataReceived] -> MATLAB Function 4/4(dataReceived)
  In1/1 -> MATLAB Function 2/2(kooVec)
  [dataDim] -> "MATLAB Function 1 "/4(dataDim)
  MATLAB Function 5/1(output) -> output/1
  MATLAB Function 4/3(readyToSend) -> MATLAB Function 5/8(output4_isReady)
  [messageToEffectuator] -> MATLAB Function 3/4(messageFromDispat)
  [massageReceived] -> "MATLAB Function 1 "/3(massageReceived)
  Delay2/1 -> MATLAB Function 4/1(prev_EffSegmentData)
  [dataDim] -> MATLAB Function 4/3(dataDim)
  MATLAB Function 4/2(output) -> MATLAB Function 5/7(output4)
  messageToEffectuator1/1 -> [axesPos]
  messageToEffectuator/1 -> [messageToEffectuator]
  messageToEffectuator2/1 -> [massageReceived]
  messageToEffectuator3/1 -> [dataDim]
  messageToEffectuator4/1 -> [dataReceived]
  Function-Call Generator/1 -> output1/1

== system EffectuatorIntegratedWithDemonstrator/udp_communication/UDP Send//Receive ==
  In1 : Inport
  function : TriggerPort  TriggerType=function-call  VariantControl=Variant
  "Real-time UDP Configuration " : ptplib/PTP UDP/Real-time UDP  Configuration   ID=1  IpAddress=192.168.5.90  SubnetMask=255.255.255.0  Gateway=0.0.0.0  EthDrv=Intel Gigabit  PciBus=5  PciSlot=0  PciFunction=0  udpID=0  MulticastList=[]  Multicast={}
      settings: SourceProductBaseCode=XP
  udp_receive : Subsystem
  udp_send : Subsystem
  messageToEffectuator2 : Outport
  messageToEffectuator3 : Outport  Port=2
  messageToEffectuator4 : Outport  Port=3
  wires:
  udp_receive/1(messageToEffectuator2) -> messageToEffectuator2/1
  In1/1 -> udp_send/1(In6)
  udp_receive/2(Out11) -> messageToEffectuator3/1
  udp_receive/3(Out12) -> messageToEffectuator4/1

== system EffectuatorIntegratedWithDemonstrator/Achse X/Segmentregler/Smooth 5Ts ==
  In1 : Inport
  Delay{,1..3} (4 alike) : Delay  DelayLength=1
  Gain : Gain  Gain=1/5
  Sum : Sum  Inputs=+++++
  Out1 : Outport  VectorParamsAs1DForOutWhenUnconnected=off
  wires:
  In1/1 -> Sum/5, Delay/1
  Delay/1 -> Sum/4, Delay1/1
  Delay1/1 -> Sum/3, Delay2/1
  Delay2/1 -> Sum/2, Delay3/1
  Delay3/1 -> Sum/1
  Sum/1 -> Gain/1
  Gain/1 -> Out1/1

== system EffectuatorIntegratedWithDemonstrator/Achse Y/Segmentregler/Smooth 5Ts ==
  In1 : Inport
  Delay{,1..3} (4 alike) : Delay  DelayLength=1
  Gain : Gain  Gain=1/5
  Sum : Sum  Inputs=+++++
  Out1 : Outport  VectorParamsAs1DForOutWhenUnconnected=off
  wires:
  Gain/1 -> Out1/1
  Sum/1 -> Gain/1
  Delay3/1 -> Sum/1
  Delay2/1 -> Delay3/1, Sum/2
  Delay1/1 -> Delay2/1, Sum/3
  Delay/1 -> Delay1/1, Sum/4
  In1/1 -> Delay/1, Sum/5

== system EffectuatorIntegratedWithDemonstrator/Achse Z/Segmentregler/Smooth 5Ts ==
  In1 : Inport
  Delay{,1..3} (4 alike) : Delay  DelayLength=1
  Gain : Gain  Gain=1/5
  Sum : Sum  Inputs=+++++
  Out1 : Outport  VectorParamsAs1DForOutWhenUnconnected=off
  wires:
  In1/1 -> Sum/5, Delay/1
  Delay/1 -> Sum/4, Delay1/1
  Delay1/1 -> Sum/3, Delay2/1
  Delay2/1 -> Sum/2, Delay3/1
  Delay3/1 -> Sum/1
  Sum/1 -> Gain/1
  Gain/1 -> Out1/1

== system EffectuatorIntegratedWithDemonstrator/Joystick Ctrl/Joystick/AchseX ==
  Inport : Inport
  Bus Selector : BusSelector  OutputSignals=signal1,signal2
  Constant : Constant  Value=50
  Data Store Write : DataStoreWrite  DataStoreName=VelOverride  SampleTime=0.5  DataStoreElements=VelOverride(1)
  Discrete-Time Integrator : DiscreteIntegrator  gainval=0.5  SampleTime=-1  LimitOutput=on  UpperSaturationLimit=1  LowerSaturationLimit=-0.75  ICPrevOutput=DiscIntNeverNeededParam  ICPrevScaledInput=DiscIntNeverNeededParam
  Idx Achse : Constant  Value=3
  Idx Knopf : Constant  Value=3
  Joystick Achse auswählen : Selector  InputPortWidth=8  IndexOptions=Index vector (port)  Indices=[3]  OutputSizes=1
  Joystick Knopf auswählen : Selector  InputPortWidth=32  IndexOptions=Index vector (port)  Indices=[3]  OutputSizes=1
  Leerweg : DeadZone  LowerValue=-0.3  UpperValue=0.3  SaturateOnIntegerOverflow=on
  Multiply : Gain  Gain=-1
  Multiply1 : Gain  Gain=50
  Multiply2 : Gain  Gain=1/100
  Product : Product
  Sum : Sum  Inputs=++|
  wires:
  Multiply1/1 -> Sum/2
  Multiply/1 -> Discrete-Time Integrator/1
  Discrete-Time Integrator/1 -> Multiply1/1
  Constant/1 -> Sum/1
  Leerweg/1 -> Multiply/1
  Joystick Achse auswählen/1 -> Product/1
  Joystick Knopf auswählen/1 -> Product/2
  Product/1 -> Leerweg/1
  Sum/1 -> Multiply2/1
  Multiply2/1 -> Data Store Write/1
  Idx Achse/1 -> Joystick Achse auswählen/2
  Idx Knopf/1 -> Joystick Knopf auswählen/2
  Bus Selector/1 -> Joystick Achse auswählen/1  "<signal1>"
  Bus Selector/2 -> Joystick Knopf auswählen/1  "<signal2>"
  Inport/1 -> Bus Selector/1

== system EffectuatorIntegratedWithDemonstrator/Joystick Ctrl/Joystick/AchseY ==
  Inport : Inport
  Bus Selector : BusSelector  OutputSignals=signal1,signal2
  Constant : Constant  Value=50
  Data Store Write : DataStoreWrite  DataStoreName=VelOverride  SampleTime=0.5  DataStoreElements=VelOverride(2)
  Discrete-Time Integrator : DiscreteIntegrator  gainval=0.5  SampleTime=-1  LimitOutput=on  UpperSaturationLimit=1  LowerSaturationLimit=-0.75  ICPrevOutput=DiscIntNeverNeededParam  ICPrevScaledInput=DiscIntNeverNeededParam
  Idx Achse : Constant  Value=3
  Idx Knopf : Constant  Value=4
  Joystick Achse auswählen : Selector  InputPortWidth=8  IndexOptions=Index vector (port)  Indices=[3]  OutputSizes=1
  Joystick Knopf auswählen : Selector  InputPortWidth=32  IndexOptions=Index vector (port)  Indices=[3]  OutputSizes=1
  Leerweg : DeadZone  LowerValue=-0.3  UpperValue=0.3  SaturateOnIntegerOverflow=on
  Multiply : Gain  Gain=-1
  Multiply1 : Gain  Gain=50
  Multiply2 : Gain  Gain=1/100
  Product : Product
  Sum : Sum  Inputs=++|
  wires:
  Inport/1 -> Bus Selector/1
  Bus Selector/2 -> Joystick Knopf auswählen/1  "<signal2>"
  Bus Selector/1 -> Joystick Achse auswählen/1  "<signal1>"
  Idx Knopf/1 -> Joystick Knopf auswählen/2
  Idx Achse/1 -> Joystick Achse auswählen/2
  Multiply2/1 -> Data Store Write/1
  Sum/1 -> Multiply2/1
  Product/1 -> Leerweg/1
  Joystick Knopf auswählen/1 -> Product/2
  Joystick Achse auswählen/1 -> Product/1
  Leerweg/1 -> Multiply/1
  Constant/1 -> Sum/1
  Discrete-Time Integrator/1 -> Multiply1/1
  Multiply/1 -> Discrete-Time Integrator/1
  Multiply1/1 -> Sum/2

== system EffectuatorIntegratedWithDemonstrator/Joystick Ctrl/Joystick/AchseZ ==
  Inport : Inport
  Bus Selector : BusSelector  OutputSignals=signal1,signal2
  Constant : Constant  Value=50
  Data Store Write : DataStoreWrite  DataStoreName=VelOverride  SampleTime=0.5  DataStoreElements=VelOverride(3)
  Discrete-Time Integrator : DiscreteIntegrator  gainval=0.5  SampleTime=-1  LimitOutput=on  UpperSaturationLimit=1  LowerSaturationLimit=-0.75  ICPrevOutput=DiscIntNeverNeededParam  ICPrevScaledInput=DiscIntNeverNeededParam
  Idx Achse : Constant  Value=3
  Idx Knopf : Constant
  Joystick Achse auswählen : Selector  InputPortWidth=8  IndexOptions=Index vector (port)  Indices=[3]  OutputSizes=1
  Joystick Knopf auswählen : Selector  InputPortWidth=32  IndexOptions=Index vector (port)  Indices=[3]  OutputSizes=1
  Leerweg : DeadZone  LowerValue=-0.3  UpperValue=0.3  SaturateOnIntegerOverflow=on
  Multiply : Gain  Gain=-1
  Multiply1 : Gain  Gain=50
  Multiply2 : Gain  Gain=1/100
  Product : Product
  Sum : Sum  Inputs=++|
  wires:
  Multiply1/1 -> Sum/2
  Multiply/1 -> Discrete-Time Integrator/1
  Discrete-Time Integrator/1 -> Multiply1/1
  Constant/1 -> Sum/1
  Leerweg/1 -> Multiply/1
  Joystick Achse auswählen/1 -> Product/1
  Joystick Knopf auswählen/1 -> Product/2
  Product/1 -> Leerweg/1
  Sum/1 -> Multiply2/1
  Multiply2/1 -> Data Store Write/1
  Idx Achse/1 -> Joystick Achse auswählen/2
  Idx Knopf/1 -> Joystick Knopf auswählen/2
  Bus Selector/1 -> Joystick Achse auswählen/1  "<signal1>"
  Bus Selector/2 -> Joystick Knopf auswählen/1  "<signal2>"
  Inport/1 -> Bus Selector/1

== system EffectuatorIntegratedWithDemonstrator/udp_communication/UDP Send//Receive/udp_receive ==
  Byte Unpack : etargetslib/Byte Unpack  dimensions={[238]}  datatypes={'int32'}  byteAlign=1
  Demux : Demux  Commented=on  Outputs=9
  Demux1 : Demux  Commented=on  Outputs=9
  Display : Display
  Display{1..10} (10 alike) : Display  Commented=on
  Display11 : Display
  MATLAB Function : MATLAB Function  TreatAsAtomicUnit=on
  Scope : Scope  Commented=on
  UDP Receive : xpcrtudplib/UDP Receive  ipAddressVal=Use host-target connection  localPort=8000  rcvWidth=238*4  rcvFmAny=off  fmAddress=192.168.5.100  rcvMulticast=off  multicastAddress={}  maxUDPQueue=8  sampleTime=-1
  UDP Receive1 : dspnetwork/UDP Receive  Commented=on  localURL='0.0.0.0'  localPort=8000  remoteURL='192.168.5.100'  remotePort=-1  recvBufferSize=8192  dims=255  signalDatatype=uint32  isComplex=off  isVarSize=on  showBlockingTime=on  blockingTime=inf  sampletime=0.01  blockPlatform=HOST
  messageToEffectuator2 : Outport
  Out11 : Outport  Port=2
  Out12 : Outport  Port=3
  wires:
  UDP Receive/2 -> Display/1
  UDP Receive/1 -> Byte Unpack/1
  Demux/4 -> ?
  Demux/3 -> ?
  Demux/2 -> ?
  Demux/1 -> ?
  UDP Receive1/1 -> Display2/1
  Demux/5 -> ?
  Demux/6 -> ?
  Demux/7 -> ?
  Demux/8 -> ?
  Demux1/8 -> Display9/1
  Demux1/7 -> Display8/1
  Demux1/6 -> Display7/1
  Demux1/5 -> Display6/1
  Demux1/1 -> Display1/1
  Demux1/2 -> Display3/1
  Demux1/3 -> Display4/1
  Demux1/4 -> Display5/1
  Demux/9 -> ?
  Demux1/9 -> Display10/1
  Byte Unpack/1 -> MATLAB Function/1(input)
  MATLAB Function/1(massageReceived) -> messageToEffectuator2/1
  MATLAB Function/2(dataDim) -> Out11/1
  MATLAB Function/3(dataReceived) -> Display11/1, Out12/1

== system EffectuatorIntegratedWithDemonstrator/udp_communication/UDP Send//Receive/udp_send ==
  In6 : Inport
  "Byte Packing " : xpcutilitieslib/Byte Packing   MaskPackedDataType=uint8  MaskUnpackedDataTypes={'int32'}  MaskAlignment=1
  Constant : Constant  Value=943*4
  Constant1 : Constant  Commented=on  Value=100
  Constant2 : Constant  Commented=on  Value=101
  Constant3 : Constant  Commented=on  Value=[1:318]  OutDataTypeStr=int32
  Display : Display  Commented=on
  Mux1 : Mux  Commented=on  Inputs=2
  Scope : Scope  Commented=on
  UDP Send : xpcrtudplib/UDP Send  ipAddressVal=Use host-target connection  localPort=8080  toAddress=192.168.5.100  toPort=8080  sampleTime=-1
      settings: SourceProductBaseCode=XP
  UDP Send1 : dspnetwork/UDP Send  Commented=on  remoteURL='192.168.5.100'  remotePort=10  localURL='0.0.0.0'  localPortSource=Specify via dialog  localPort=8000  sendBufferSize=8192  sampletime=-1  blockPlatform=HOST  separateLengthPort=0
  wires:
  Constant/1 -> UDP Send/2
  "Byte Packing "/1 -> UDP Send/1
  Mux1/1 -> UDP Send1/1
  Constant1/1 -> Mux1/1
  Constant2/1 -> Mux1/2
  In6/1 -> "Byte Packing "/1
